simulink model "Problema8_2"  (R2018b)
settings: Solver=VariableStepAuto  StartTime=0.0  StopTime=25  RelTol=1e-3
values from neighbouring files (symbols this model uses):
  A = [ -3 0; 1 0 ]    [Problema8_2.m]
  B = [ 1; 0]    [Problema8_2.m]
  C = [ 0 1 ]    [Problema8_2.m]
  Ca = [1 0;0 1]    [Problema8_2.m]
  D = 0    [Problema8_2.m]
  Da = [0;0]    [Problema8_2.m]
  h = 0.2    [Problema8_2.m]
  L = [0 1] * inv(Wc) * (phi^2 + p1 * phi + p2 * eye(2))    [Problema8_2.m]
  Lc = ganho_dc/( C * inv(eye(2) - phi_cl ) * gama )    [Problema8_2.m]
  x0 = [ 0 0 ]'    [Problema8_2.m]
settings Model: Creator=Asus  LastModifiedBy=fredericovaz
settings SFSimCC: SimUseLocalCustomCode=off
settings RTWCC: RTWUseLocalCustomCode=off
settings CodeAppCC: StateflowObjectComments=on

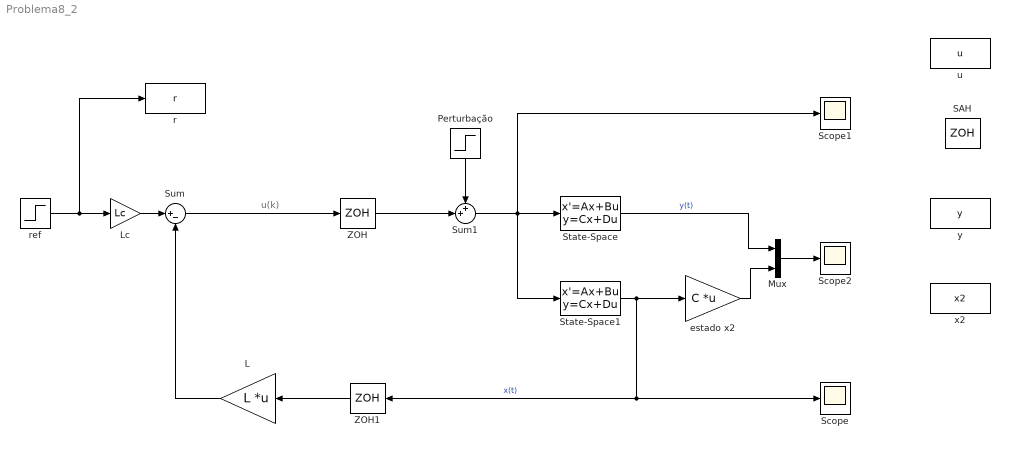
== system Problema8_2 ==
  note: u(k)
  L : Gain  Gain=L  Multiplication=Matrix(K*u) (u vector)
  Lc : Gain  Gain=Lc
  Mux : Mux  Inputs=2
  Perturbação : Step  Time=15  After=0.3  SampleTime=0
  SAH : ZeroOrderHold  SampleTime=h
  Scope : Scope
  Scope1 : Scope
  Scope2 : Scope
  State-Space : StateSpace  A=A  B=B  C=C  D=D  InitialCondition=x0
  State-Space1 : StateSpace  A=A  B=B  C=Ca  D=Da  InitialCondition=x0
  Sum : Sum  Inputs=|+-
  Sum1 : Sum  Inputs=++|
  ZOH : ZeroOrderHold  SampleTime=h
  ZOH1 : ZeroOrderHold  SampleTime=h
  "estado x2 " : Gain  Gain=C  Multiplication=Matrix(K*u) (u vector)
  r : ToWorkspace  VariableName=r  SaveFormat=Structure With Time  SampleTime=-1
  "ref " : Step  Time=5  After=0.4  SampleTime=0
  u : ToWorkspace  VariableName=u  SaveFormat=Structure With Time  SampleTime=-1
  x2 : ToWorkspace  VariableName=x2  SaveFormat=Structure With Time  SampleTime=-1
  y : ToWorkspace  VariableName=y  SaveFormat=Structure With Time  SampleTime=-1
  wires:
  ZOH/1 -> Sum1/2
  L/1 -> Sum/2
  Sum1/1 -> Scope1/1, State-Space1/1, State-Space/1
  Lc/1 -> Sum/1
  "ref "/1 -> r/1, Lc/1
  Sum/1 -> ZOH/1
  ZOH1/1 -> L/1
  Perturbação/1 -> Sum1/1
  State-Space1/1 -> Scope/1, ZOH1/1, "estado x2 "/1  "x(t)"
  Mux/1 -> Scope2/1
  "estado x2 "/1 -> Mux/2
  State-Space/1 -> Mux/1  "y(t)"
